simulink model "circuit"  (R2017a)
settings: Solver=VariableStepAuto  StartTime=0.0  StopTime=10.0  RelTol=1e-3
libraries: pe_lib x6
settings Model: Creator=k1506456  LastModifiedBy=k1506456

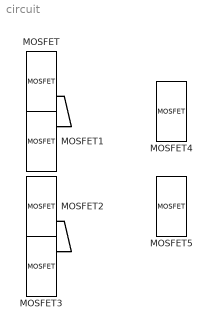
== system circuit ==
  MOSFET{,1..5} (6 alike) : pe_lib/Semiconductors/Fundamental Components/MOSFET  Rds=0.01 Ohm  Goff=1e-6 1/Ohm  Vth=2 V  diode_param=2  diode_Vf=0.8 V  diode_Ron=0.001 Ohm  diode_Goff=1e-5 1/Ohm  diode_C=5e-8 F  diode_iRM=-235 A  diode_iF=300 A  diode_idot=-50 A/us  diode_trr_param=1  diode_trr_factor=3  diode_trr=15 us  diode_Qrr=1.5e+3 s*uA  thermal_loss_option=2  Voff=300 V  Tau=1e-4 s  Tj=[ 298.15 398.15 ] K  Iout_scalar=600 A  Eon_scalar=0.02286 J  Eoff_scalar=0.01714 J  Von_scalar=2.7 V  Iout_data=[ 0 10 50 100 200 400 600 ] A  Eon_data=[ 0 2.9e-4 0.00143 0.00286 0.00571 0.01314 0.02286; 0 5.7e-4 0.00263 0.00514 0.01029 0.02057 0.03029 ] J  Eoff_data=[ 0 2.1e-4 0.00107 0.00214 0.00429 0.009859999999999999 0.01714; 0 4.3e-4 0.00197 0.00386 0.00771 0.01543 0.02271 ] J  Von_data=[ 0 1.1 1.3 1.45 1.75 2.25 2.7; 0 1 1.15 1.35 1.7 2.35 3 ] V
      settings: SourceProductName=Simscape Power Systems  SourceProductBaseCode=PS
  connections:
  MOSFET1/RConn2 -- MOSFET/RConn2
  MOSFET3/RConn2 -- MOSFET2/RConn2
